simulink model "Aufiero_detumbling"  (R2021a)
settings: Solver=VariableStepAuto  StartTime=0.0  StopTime=250  FixedStep=1/262  RelTol=1e-3
settings Model: Creator=daniele.leuteri  LastModifiedBy=aufie
settings SolverCC: AlgebraicLoopSolver=TrustRegion
settings DebuggingCC: SFMachineParentedDataDiag=warning
settings SFSimCC: CustomCodeUndefinedFunction=UseInterfaceOnly

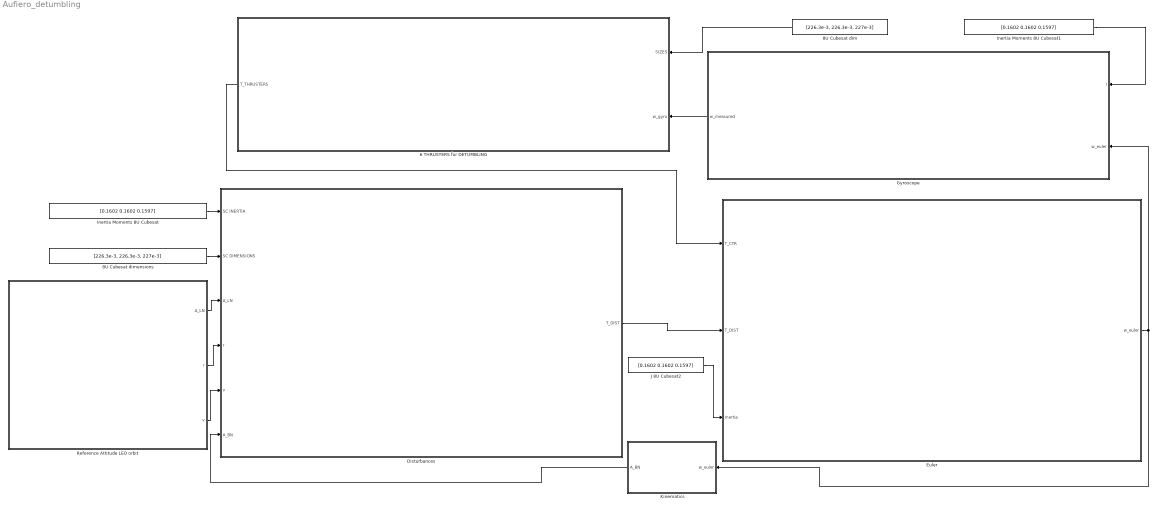
== system Aufiero_detumbling ==
  6 THRUSTERS for DETUMBLING : Subsystem
  8U Cubesat dim : Constant  Value=[226.3e-3, 226.3e-3, 227e-3]
  8U Cubesat dimensions : Constant  Value=[226.3e-3, 226.3e-3, 227e-3]
  Disturbances : Subsystem
  Euler : Subsystem
  Gyroscope : Subsystem
  Inertia Moments 8U Cubesat : Constant  Value=[0.1602 0.1602 0.1597]
  Inertia Moments 8U Cubesat1 : Constant  Value=[0.1602 0.1602 0.1597]
  J 8U Cubesat2 : Constant  Value=[0.1602 0.1602 0.1597]
  Kinematics : Subsystem
  Reference Attitude LEO orbit : Subsystem
  wires:
  8U Cubesat dimensions/1 -> Disturbances/2(SC DIMENSIONS)
  Reference Attitude LEO orbit/1(A_LN) -> Disturbances/3(A_LN)
  Reference Attitude LEO orbit/2(r) -> Disturbances/4(r)
  Reference Attitude LEO orbit/3(v) -> Disturbances/5(v)
  Inertia Moments 8U Cubesat/1 -> Disturbances/1(SC INERTIA)
  Kinematics/1(A_BN) -> Disturbances/6(A_BN)
  J 8U Cubesat2/1 -> Euler/3(Inertia)
  Disturbances/1(T_DIST) -> Euler/2(T_DIST)
  Inertia Moments 8U Cubesat1/1 -> Gyroscope/1(I)
  8U Cubesat dim/1 -> 6 THRUSTERS for DETUMBLING/1(SIZES)
  6 THRUSTERS for DETUMBLING/1(T_THRUSTERS) -> Euler/1(T_CTR)
  Gyroscope/1(w_measured) -> 6 THRUSTERS for DETUMBLING/2(w_gyro)
  Euler/1(w_euler) -> Kinematics/1(w_euler), Gyroscope/2(w_euler)

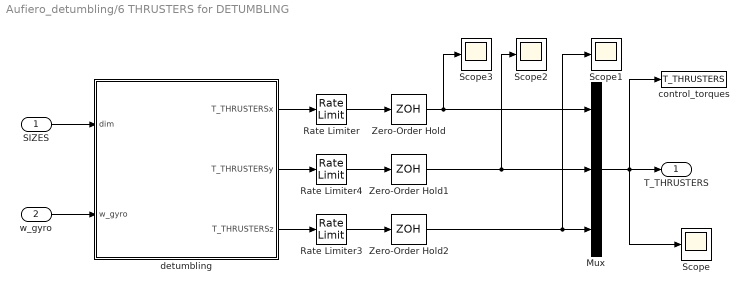
== system Aufiero_detumbling/6 THRUSTERS for DETUMBLING ==
  SIZES : Inport
  w_gyro : Inport  Port=2
  Mux : Mux  Inputs=3
  Rate Limiter : RateLimiter  RisingSlewLimit=1/0.1  FallingSlewLimit=-1/0.5  SampleTimeMode=inherited
  Rate Limiter3 : RateLimiter  RisingSlewLimit=1/0.1  FallingSlewLimit=-1/0.5  SampleTimeMode=inherited
  Rate Limiter4 : RateLimiter  RisingSlewLimit=1/0.1  FallingSlewLimit=-1/0.5  SampleTimeMode=inherited
  Scope{,1..3} (4 alike) : Scope
  Zero-Order Hold : ZeroOrderHold  SampleTime=0.05e-03
  Zero-Order Hold1 : ZeroOrderHold  SampleTime=0.05e-03
  Zero-Order Hold2 : ZeroOrderHold  SampleTime=0.05e-03
  control_torques : ToWorkspace  VariableName=T_THRUSTERS  SaveFormat=Timeseries  SampleTime=-1
  detumbling : MATLAB Function  TreatAsAtomicUnit=on
  T_THRUSTERS : Outport  VectorParamsAs1DForOutWhenUnconnected=off
  wires:
  SIZES/1 -> detumbling/1(dim)
  w_gyro/1 -> detumbling/2(w_gyro)
  Zero-Order Hold/1 -> Mux/1, Scope3/1
  Zero-Order Hold1/1 -> Mux/2, Scope2/1
  Zero-Order Hold2/1 -> Scope1/1, Mux/3
  Mux/1 -> control_torques/1, T_THRUSTERS/1, Scope/1
  detumbling/2(T_THRUSTERSy) -> Rate Limiter4/1
  detumbling/1(T_THRUSTERSx) -> Rate Limiter/1
  detumbling/3(T_THRUSTERSz) -> Rate Limiter3/1
  Rate Limiter/1 -> Zero-Order Hold/1
  Rate Limiter4/1 -> Zero-Order Hold1/1
  Rate Limiter3/1 -> Zero-Order Hold2/1

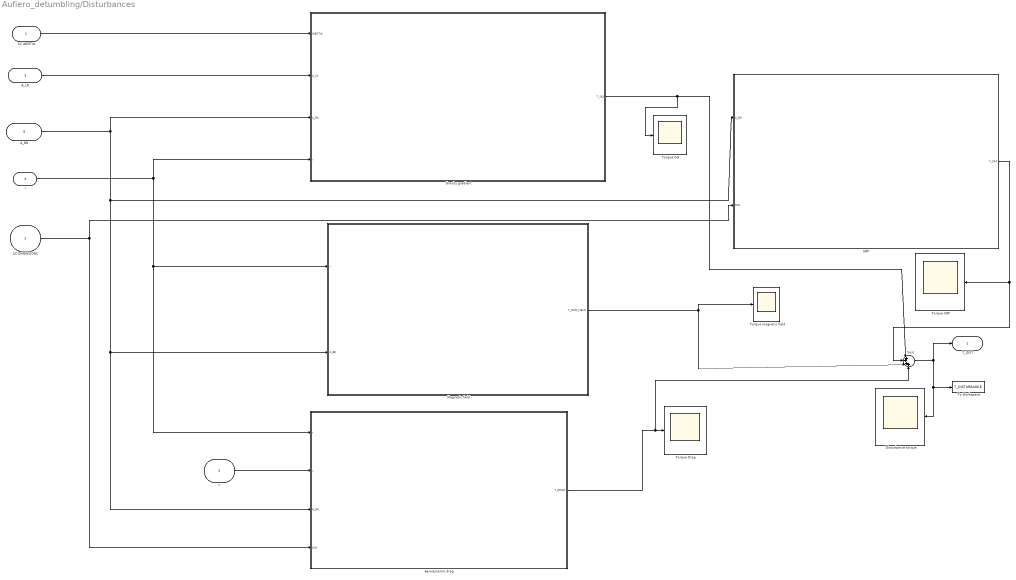
== system Aufiero_detumbling/Disturbances ==
  SC INERTIA : Inport
  SC DIMENSIONS : Inport  Port=2
  A_LN : Inport  Port=3
  r : Inport  Port=4
  v : Inport  Port=5
  A_BN : Inport  Port=6
  Aerodynamic drag : Subsystem
  Disturbance torque : Scope
  Gravity gradient : Subsystem
  Magnetic field : Subsystem
  SRP : Subsystem
  Sum : Sum  Inputs=|++++
  To Workspace : ToWorkspace  VariableName=T_DISTURBANCE  SaveFormat=Timeseries  SampleTime=-1
  Torque Drag : Scope
  Torque GG : Scope
  Torque SRP : Scope
  Torque magnetic field : Scope
  T_DIST : Outport  VectorParamsAs1DForOutWhenUnconnected=off
  wires:
  r/1 -> Gravity gradient/4(r), Aerodynamic drag/1(r), Magnetic field/1(r)
  v/1 -> Aerodynamic drag/2(v)
  A_BN/1 -> Gravity gradient/3(A_BN), Aerodynamic drag/3(A_BN), Magnetic field/2(A_BN), SRP/1(A_BN)
  SC DIMENSIONS/1 -> SRP/2(DIM), Aerodynamic drag/4(DIM)
  SC INERTIA/1 -> Gravity gradient/1(INERTIA)
  A_LN/1 -> Gravity gradient/2(A_LN)
  Gravity gradient/1(T_GG) -> Sum/1, Torque GG/1
  SRP/1(T_SRP) -> Sum/2, Torque SRP/1
  Aerodynamic drag/1(T_DRAG) -> Sum/4, Torque Drag/1
  Magnetic field/1(T_MAG_FIELD) -> Torque magnetic field/1, Sum/3
  Sum/1 -> Disturbance torque/1, To Workspace/1, T_DIST/1

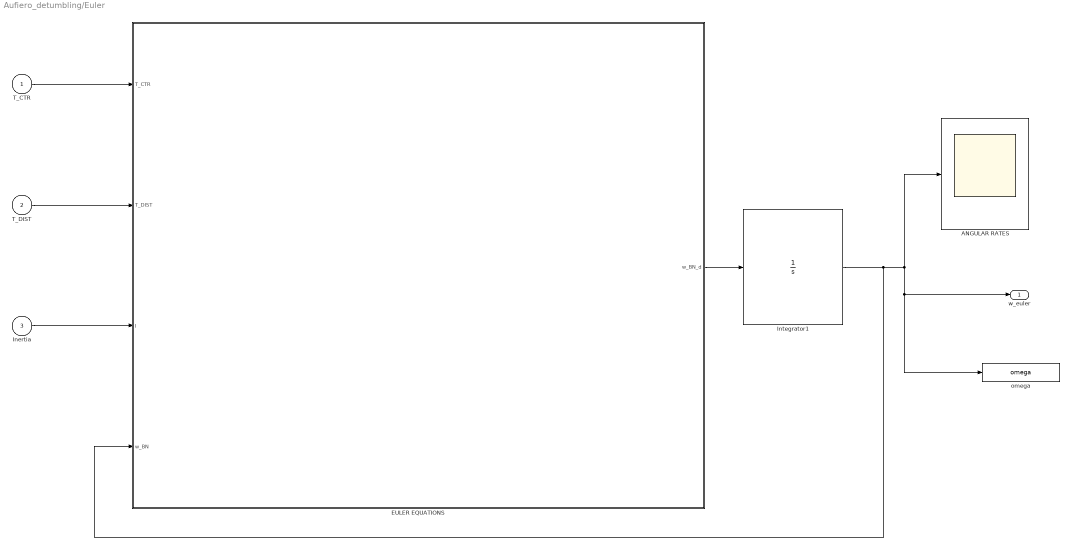
== system Aufiero_detumbling/Euler ==
  T_CTR : Inport
  T_DIST : Inport  Port=2
  Inertia : Inport  Port=3
  ANGULAR RATES : Scope
  EULER EQUATIONS : MATLAB Function  TreatAsAtomicUnit=on
  Integrator1 : Integrator  InitialCondition=[0.1 0.1 0.1]
  omega : ToWorkspace  VariableName=omega  SaveFormat=Timeseries  SampleTime=-1
  w_euler : Outport  VectorParamsAs1DForOutWhenUnconnected=off
  wires:
  T_CTR/1 -> EULER EQUATIONS/1(T_CTR)
  Inertia/1 -> EULER EQUATIONS/3(I)
  EULER EQUATIONS/1(w_BN_d) -> Integrator1/1
  T_DIST/1 -> EULER EQUATIONS/2(T_DIST)
  Integrator1/1 -> omega/1, w_euler/1, ANGULAR RATES/1, EULER EQUATIONS/4(w_BN)

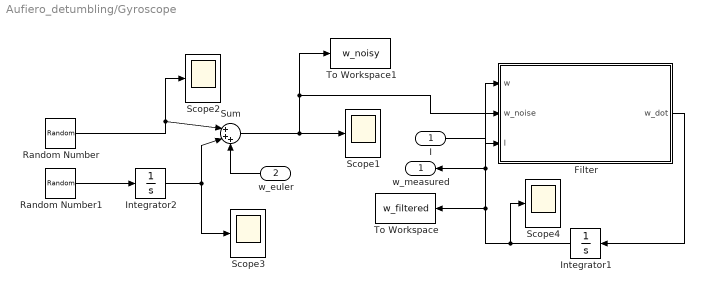
== system Aufiero_detumbling/Gyroscope ==
  I : Inport
  w_euler : Inport  Port=2
  "Filter " : MATLAB Function  TreatAsAtomicUnit=on
  Integrator1 : Integrator  InitialCondition=[0.1 0.1 0.1]
  Integrator2 : Integrator
  Random Number : RandomNumber  Variance=(0.15*pi/180/3600)*sqrt(1/262)  SampleTime=1/262
  Random Number1 : RandomNumber  Variance=(0.3*pi/180/3600)*sqrt(1/262)  SampleTime=1/262
  Scope{1..4} (4 alike) : Scope
  Sum : Sum  Inputs=|+++
  To Workspace : ToWorkspace  VariableName=w_filtered  SaveFormat=Timeseries  SampleTime=-1
  To Workspace1 : ToWorkspace  VariableName=w_noisy  SaveFormat=Timeseries  SampleTime=-1
  w_measured : Outport  VectorParamsAs1DForOutWhenUnconnected=off
  wires:
  Integrator1/1 -> Scope4/1, w_measured/1, "Filter "/1(w), To Workspace/1
  Random Number1/1 -> Integrator2/1
  Sum/1 -> To Workspace1/1, "Filter "/2(w_noise), Scope1/1
  Integrator2/1 -> Scope3/1, Sum/2
  Random Number/1 -> Scope2/1, Sum/1
  "Filter "/1(w_dot) -> Integrator1/1
  w_euler/1 -> Sum/3
  I/1 -> "Filter "/3(I)

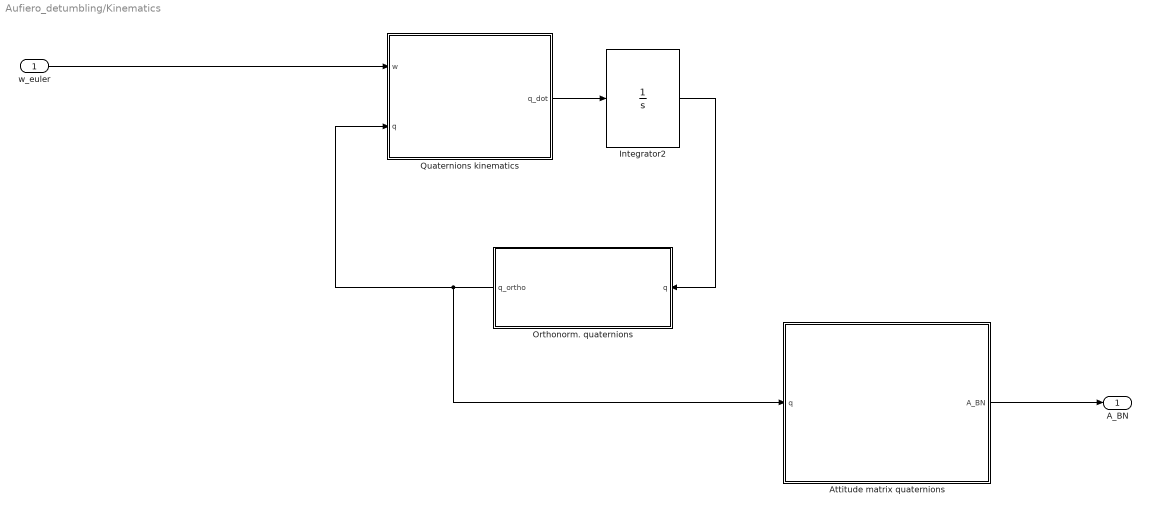
== system Aufiero_detumbling/Kinematics ==
  w_euler : Inport
  Attitude matrix quaternions : MATLAB Function  TreatAsAtomicUnit=on
  Integrator2 : Integrator  InitialCondition=[0 1/sqrt(3) 1/sqrt(3) 1/sqrt(3)]
  "Orthonorm. quaternions " : MATLAB Function  TreatAsAtomicUnit=on
  "Quaternions kinematics " : MATLAB Function  TreatAsAtomicUnit=on
  A_BN : Outport  VectorParamsAs1DForOutWhenUnconnected=off
  wires:
  w_euler/1 -> "Quaternions kinematics "/1(w)
  "Orthonorm. quaternions "/1(q_ortho) -> Attitude matrix quaternions/1(q), "Quaternions kinematics "/2(q)
  "Quaternions kinematics "/1(q_dot) -> Integrator2/1
  Attitude matrix quaternions/1(A_BN) -> A_BN/1
  Integrator2/1 -> "Orthonorm. quaternions "/1(q)

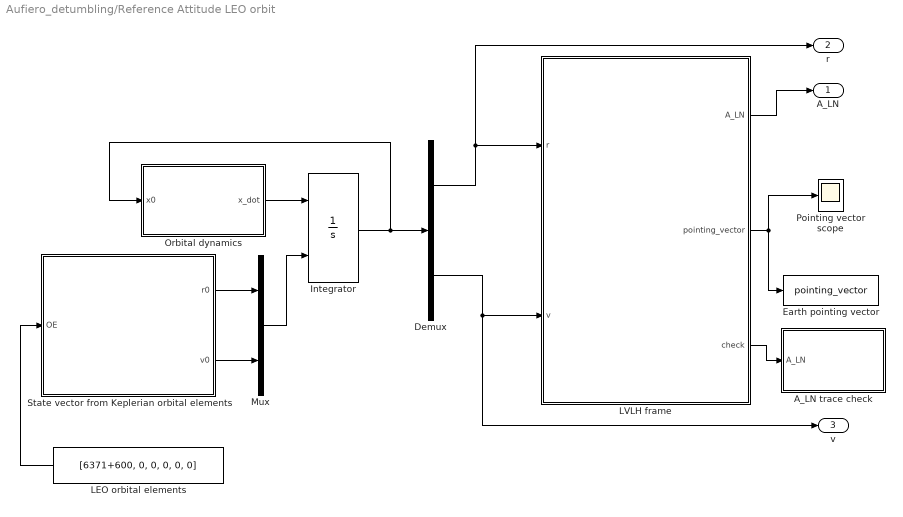
== system Aufiero_detumbling/Reference Attitude LEO orbit ==
  A_LN trace check : Subsystem
  Demux : Demux  Outputs=2
  Earth pointing vector : ToWorkspace  VariableName=pointing_vector  SampleTime=-1
  Integrator : Integrator  InitialConditionSource=external
  "LEO orbital elements " : Constant  Value=[6371+600, 0, 0, 0, 0, 0]
  LVLH frame : MATLAB Function  TreatAsAtomicUnit=on
  Mux : Mux  Inputs=2
  Orbital dynamics : MATLAB Function  TreatAsAtomicUnit=on
  Pointing vector scope : Scope
  State vector from Keplerian orbital elements : MATLAB Function  TreatAsAtomicUnit=on
  A_LN : Outport  VectorParamsAs1DForOutWhenUnconnected=off
  r : Outport  Port=2  VectorParamsAs1DForOutWhenUnconnected=off
  v : Outport  Port=3  VectorParamsAs1DForOutWhenUnconnected=off
  wires:
  LVLH frame/1(A_LN) -> A_LN/1
  Integrator/1 -> Demux/1, Orbital dynamics/1(x0)
  State vector from Keplerian orbital elements/2(v0) -> Mux/2
  Demux/2 -> v/1, LVLH frame/2(v)
  Demux/1 -> r/1, LVLH frame/1(r)
  Mux/1 -> Integrator/2
  Orbital dynamics/1(x_dot) -> Integrator/1
  State vector from Keplerian orbital elements/1(r0) -> Mux/1
  "LEO orbital elements "/1 -> State vector from Keplerian orbital elements/1(OE)
  LVLH frame/2(pointing_vector) -> Earth pointing vector/1, Pointing vector scope/1
  LVLH frame/3(check) -> A_LN trace check/1(A_LN)

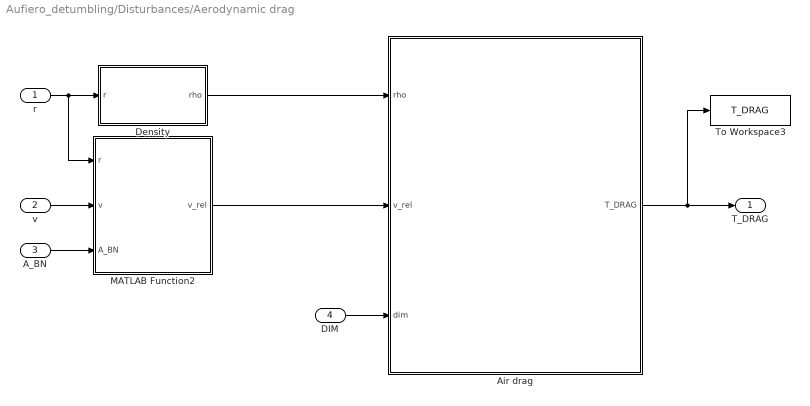
== system Aufiero_detumbling/Disturbances/Aerodynamic drag ==
  r : Inport
  v : Inport  Port=2
  A_BN : Inport  Port=3
  DIM : Inport  Port=4
  Air drag : MATLAB Function  TreatAsAtomicUnit=on
  Density : MATLAB Function  TreatAsAtomicUnit=on
  MATLAB Function2 : MATLAB Function  TreatAsAtomicUnit=on
  To Workspace3 : ToWorkspace  VariableName=T_DRAG  SaveFormat=Timeseries  SampleTime=-1
  T_DRAG : Outport  VectorParamsAs1DForOutWhenUnconnected=off
  wires:
  MATLAB Function2/1(v_rel) -> Air drag/2(v_rel)
  A_BN/1 -> MATLAB Function2/3(A_BN)
  Density/1(rho) -> Air drag/1(rho)
  v/1 -> MATLAB Function2/2(v)
  r/1 -> MATLAB Function2/1(r), Density/1(r)
  DIM/1 -> Air drag/3(dim)
  Air drag/1(T_DRAG) -> T_DRAG/1, To Workspace3/1

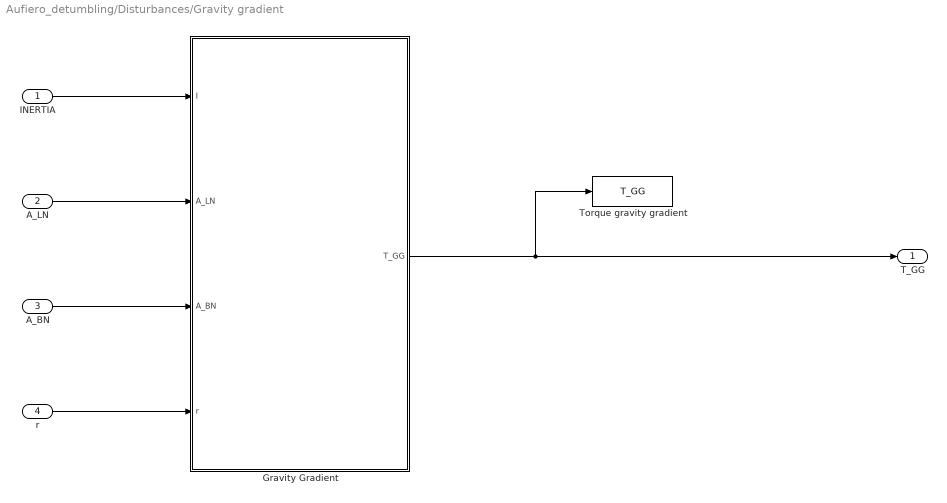
== system Aufiero_detumbling/Disturbances/Gravity gradient ==
  INERTIA : Inport
  A_LN : Inport  Port=2
  A_BN : Inport  Port=3
  r : Inport  Port=4
  Gravity Gradient : MATLAB Function  TreatAsAtomicUnit=on
  Torque gravity gradient : ToWorkspace  VariableName=T_GG  SaveFormat=Timeseries  SampleTime=-1
  T_GG : Outport  VectorParamsAs1DForOutWhenUnconnected=off
  wires:
  Gravity Gradient/1(T_GG) -> T_GG/1, Torque gravity gradient/1
  INERTIA/1 -> Gravity Gradient/1(I)
  A_LN/1 -> Gravity Gradient/2(A_LN)
  A_BN/1 -> Gravity Gradient/3(A_BN)
  r/1 -> Gravity Gradient/4(r)

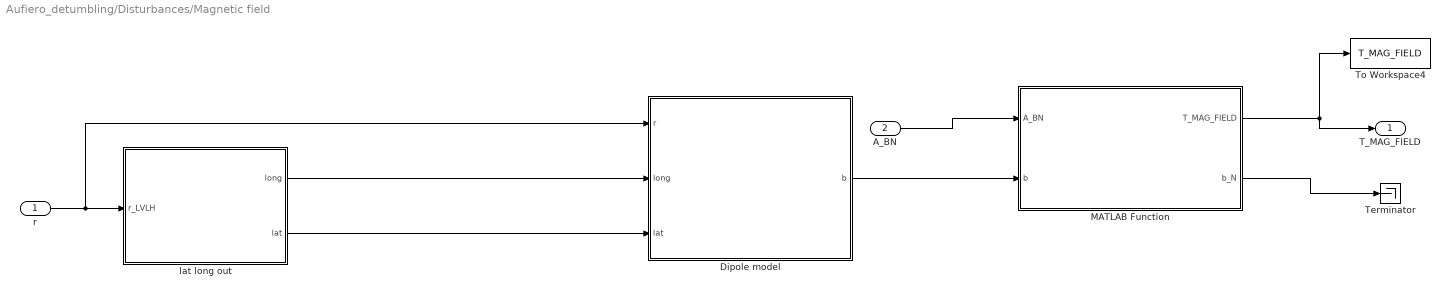
== system Aufiero_detumbling/Disturbances/Magnetic field ==
  r : Inport
  A_BN : Inport  Port=2
  Dipole model : MATLAB Function  TreatAsAtomicUnit=on
  MATLAB Function : MATLAB Function  TreatAsAtomicUnit=on
  Terminator : Terminator
  To Workspace4 : ToWorkspace  VariableName=T_MAG_FIELD  SaveFormat=Timeseries  SampleTime=-1
  "lat long out " : MATLAB Function  TreatAsAtomicUnit=on
  T_MAG_FIELD : Outport  VectorParamsAs1DForOutWhenUnconnected=off
  wires:
  r/1 -> Dipole model/1(r), "lat long out "/1(r_LVLH)
  A_BN/1 -> MATLAB Function/1(A_BN)
  Dipole model/1(b) -> MATLAB Function/2(b)
  MATLAB Function/1(T_MAG_FIELD) -> T_MAG_FIELD/1, To Workspace4/1
  MATLAB Function/2(b_N) -> Terminator/1
  "lat long out "/1(long) -> Dipole model/2(long)
  "lat long out "/2(lat) -> Dipole model/3(lat)

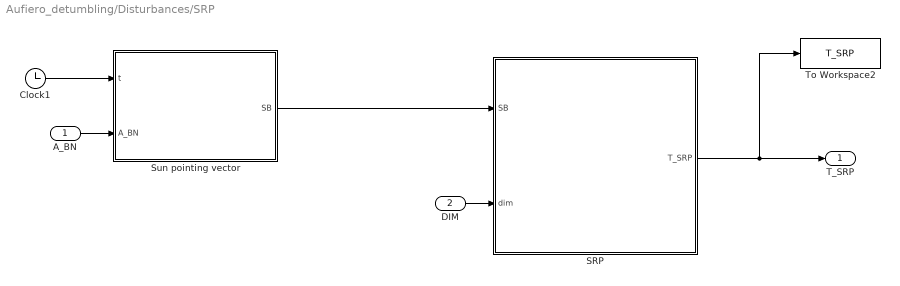
== system Aufiero_detumbling/Disturbances/SRP ==
  A_BN : Inport
  DIM : Inport  Port=2
  Clock1 : Clock
  SRP : MATLAB Function  TreatAsAtomicUnit=on
  Sun pointing vector : MATLAB Function  TreatAsAtomicUnit=on
  To Workspace2 : ToWorkspace  VariableName=T_SRP  SaveFormat=Timeseries  SampleTime=-1
  T_SRP : Outport  VectorParamsAs1DForOutWhenUnconnected=off
  wires:
  A_BN/1 -> Sun pointing vector/2(A_BN)
  DIM/1 -> SRP/2(dim)
  SRP/1(T_SRP) -> T_SRP/1, To Workspace2/1
  Clock1/1 -> Sun pointing vector/1(t)
  Sun pointing vector/1(SB) -> SRP/1(SB)

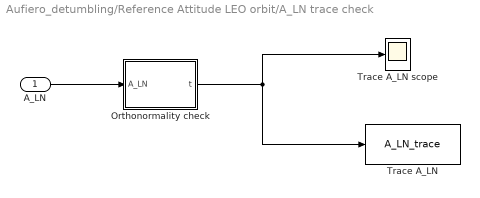
== system Aufiero_detumbling/Reference Attitude LEO orbit/A_LN trace check ==
  A_LN : Inport
  Orthonormality check : MATLAB Function  TreatAsAtomicUnit=on
  Trace A_LN : ToWorkspace  VariableName=A_LN_trace  SaveFormat=Timeseries  SampleTime=-1
  Trace A_LN scope : Scope
  wires:
  A_LN/1 -> Orthonormality check/1(A_LN)
  Orthonormality check/1(t) -> Trace A_LN scope/1, Trace A_LN/1

== matlab function Aufiero_detumbling/Disturbances/Aerodynamic drag/Density ==
  data: r input; rho output
function rho = exp_density_model(r)

r = norm(r);
h = (r - 6371000)*10^-3; % actual height [km]

if          h>=0 && h<25
            h_0 =   0; rho_0 =  1.225    ; H =   7.249;
    
elseif      h>=25 && h<30
            h_0 =   25; rho_0 = 3.899e-2 ; H =   6.349;
            
elseif      h>=30 && h<40
            h_0 =   30; rho_0 = 1.774e-2 ; H =   6.682;
                       
elseif      h>=40 && h<50
            h_0 =   40; rho_0 = 3.972e-3 ; H =   7.554;
            
elseif      h>=50 && h<60
            h_0 =   50; rho_0 = 1.057e-3 ; H =   8.382;
            
elseif      h>=60 && h<70
            h_0 =   60; rho_0 = 3.206e-4 ; H =   7.714;
            
elseif      h>=70 && h<80
            h_0 =   70; rho_0 = 8.770e-5 ; H =   6.549;

elseif      h>=80 && h<90
            h_0 =   80; rho_0 = 1.905e-5 ; H =   5.799;
            
elseif      h>=90 && h<100
            h_0 =   90; rho_0 = 3.396e-6 ; H =   5.382;
            
elseif      h>=100 && h<110
            h_0 =  100; rho_0 = 5.297e-7 ; H =   5.877;            
            
elseif      h>=110 && h<120
            h_0 =  110; rho_0 = 9.661e-8 ; H =   7.263;
            
elseif      h>=120 && h<130
            h_0 =  120; rho_0 = 2.438e-8 ; H =   9.473;           
            
elseif      h>=130 && h<140
            h_0 =  130; rho_0 = 8.484e-9 ; H =  12.636;
            
elseif      h>=140 && h<150
            h_0 =  140; rho_0 = 3.845e-9 ; H =  16.149;            
            
elseif      h>=150 && h<180
            h_0 =  150; rho_0 = 2.070e-9 ; H =  22.523;            
            
elseif      h>=180 && h<200
            h_0 =  180; rho_0 = 5.464e-10; H =  29.740;
            
elseif      h>=200 && h<250
            h_0 =  200; rho_0 = 2.789e-10; H =  37.105;            
            
elseif      h>=250 && h<300
            h_0 =  250; rho_0 = 7.248e-11; H =  45.546;            
            
elseif      h>=300 && h<350
            h_0 =  300; rho_0 = 2.418e-11; H =  53.628;
            
elseif      h>=350 && h<400
            h_0 =  350; rho_0 = 9.158e-12; H =  53.298;            
            
elseif      h>=400 && h<450
            h_0 =  400; rho_0 = 3.725e-12; H =  58.515;
            
elseif      h>=450 && h<500
            h_0 =  450; rho_0 = 1.585e-12; H =  60.828;
            
elseif      h>=500 && h<600
            h_0 =  500; rho_0 = 6.967e-13; H =  63.822;
            
elseif      h>=600 && h<700
            h_0 =  600; rho_0 = 1.454e-13; H =  71.835;            
            
elseif      h>=700 && h<800
            h_0 =  700; rho_0 = 3.614e-14; H =  88.667;            
            
elseif      h>=800 && h<900
            h_0 =  800; rho_0 = 1.170e-14; H = 124.64;
            
elseif      h>=900 && h<1000
            h_0 =  900; rho_0 = 5.245e-15; H = 181.05;                       
         
else      
            h_0 = 1000; rho_0 = 3.019e-15; H = 268.00;
            
end


rho = rho_0*exp(-(h-h_0)/H);

== matlab function Aufiero_detumbling/Disturbances/Aerodynamic drag/MATLAB Function2 ==
  data: r input; v_rel output; v input; A_BN input
function v_rel = relative_velocity(r,v,A_BN)

 % relative velocity between air and spacecraft
 
 v_rel = zeros (3,1);
 
 
 v_rel(1) = v(1) + 0.000072921*r(2);
 v_rel(2) = v(2) - 0.000072921*r(1);
 v_rel(3) = v(3);
 
 v_rel = A_BN * v_rel;
 
end

== matlab function Aufiero_detumbling/Euler/EULER EQUATIONS ==
  data: T_CTR input; T_DIST input; I input; w_BN input; w_BN_d output
function w_BN_d = euler (T_CTR, T_DIST, I, w_BN)

% EULER EQUATIONS INLCUDING DISTURBANCES AND CONTROL TORQUES

w_BN_d = zeros (1,3);

% DISTURBANCES + CONTROL TORQUE
w_BN_d(1) = (I(2)-I(3))/I(1)*w_BN(2)*w_BN(3) + T_DIST(1)/I(1) + T_CTR(1)/I(1);
w_BN_d(2) = (I(3)-I(1))/I(2)*w_BN(1)*w_BN(3) + T_DIST(2)/I(2) + T_CTR(2)/I(2);
w_BN_d(3) = (I(1)-I(2))/I(3)*w_BN(1)*w_BN(2) + T_DIST(3)/I(3) + T_CTR(3)/I(3);


w_BN_d = [w_BN_d(1) w_BN_d(2) w_BN_d(3)];


end

== matlab function Aufiero_detumbling/Kinematics/Attitude matrix quaternions ==
  data: q input; A_BN output
%function [A, ea_q] = quat_to_DCM(q)
function A_BN  = quat_to_DCM(q)

%% Elements of the A matrix as f(q)

A11 = q(1)^2 - q(2)^2 - q(3)^2 + q(4)^2;
A12 = 2*(q(1)*q(2) + q(3)*q(4));
A13 = 2*(q(1)*q(3) - q(2)*q(4));

A21 = 2*(q(1)*q(2) - q(3)*q(4));
A22 = -q(1)^2 + q(2)^2 - q(3)^2 + q(4)^2;
A23 = 2*(q(2)*q(3) + q(1)*q(4));

A31 = 2*(q(1)*q(3) + q(2)*q(4));
A32 = 2*(q(2)*q(3) - q(1)*q(4));
A33 = -q(1)^2 - q(2)^2 + q(3)^2 + q(4)^2;

A_BN = [ A11 A12 A13
      A21 A22 A23
      A31 A32 A33  ];

% %% New Euler Angles
% 
% phi = acosd(A(3,3));
% theta = -atand(A(3,1)/A(3,2));
% psi = atand(A(1,3)/A(2,3));
% 
% ea_q = [phi theta psi];

end

== matlab function Aufiero_detumbling/Disturbances/Magnetic field/Dipole model ==
  data: r input; long input; b output; lat input
function b = dipole_model(r, long, lat)

n_pole = [cos(80.37*pi/180)*cos(-72.62*pi/180);
          cos(80.37*pi/180)*sin(-72.62*pi/180);
                sin(80.37*pi/180)];
m_hat = -n_pole;

% Gaussian coefficients - IGRF 2015
g10 = -29442.0; %[nT]
g11 = -1501.0; %[nT]
h11 = 4797.1; %[nT]
H0 = sqrt(g10^2 + g11^2 + h11^2);
R_earth = 6371;

r_unit = [cos(lat*pi/180)*cos(long*pi/180);
    cos(lat*pi/180)*sin(long*pi/180);
    sin(lat*pi/180)];

b = (R_earth/norm(r))^3*H0*(3*dot(m_hat,r_unit)*r_unit - m_hat); %[nT]

end

== matlab function Aufiero_detumbling/Kinematics/Orthonorm. quaternions  ==
  data: q input; q_ortho output
function q_ortho = orho_quat(q)

Q1 = q(1)^2;
Q2 = q(2)^2;
Q3 = q(3)^2;
Q4 = q(4)^2;

Q = Q1 + Q2 + Q3 + Q4;

q_ortho = q/Q;

== matlab function Aufiero_detumbling/Kinematics/Quaternions kinematics  ==
  data: w input; q_dot output; q input
function q_dot = fcn(w, q)
% The input quaternions are already the orthonormalized ones

W = [   0   w(3)    -w(2)   w(1); 
      -w(3)  0       w(1)   w(2); 
       w(2) -w(1)     0     w(3); 
      -w(1) -w(2)   -w(3)    0   ];

q_dot = 0.5 * (W * q);

== matlab function Aufiero_detumbling/Disturbances/SRP/Sun pointing vector ==
  data: t input; SB output; A_BN input
function SB = sun_pointing(t, A_BN)

n = 2*pi/(365.25*3600*24); % Mean motion 
t0 = 0; % Initial time for the simulation 
eps = 23.45*pi/180; % Ecliptic inclination

% Sun pointing vector in inertial sun-centered reference frame
SN = [cos(n*t+t0); sin(n*t+t0)*cos(eps); sin(n*t+t0)*sin(eps)];

% Sun pointing vector in body frame
SB = A_BN * SN;

== matlab function Aufiero_detumbling/Disturbances/Magnetic field/lat long out  ==
  data: r_LVLH input; long output; lat output
function [long, lat] = ra_dec_from_r(r_LVLH)
% This function calculates the right ascension and the declination
% from the geocentric equatorial position vector.
%
% INPUT
%   r       position vector in ECI frame        [km]        [1x3]
%
% OUTPUT
%   ra      right ascension                     [deg]
%   dec     declination                         [deg]
%
%   Verified by Daniele Leuteri Costanzo

%% CALCULATE DIRECTION COSINES
l = r_LVLH(1)/norm(r_LVLH);
m = r_LVLH(2)/norm(r_LVLH);
n = r_LVLH(3)/norm(r_LVLH);

%% CALCULATE DECLINATION

lat = asind(n);

%% CALCULATE RIGHT ASCENSION

    if m > 0
        long = acosd(l/cosd(lat));
    else
        long = 360 - acosd(l/cosd(lat));
    end
end

== matlab function Aufiero_detumbling/Disturbances/Magnetic field/MATLAB Function ==
  data: A_BN input; T_MAG_FIELD output; b input; b_N output
function [T_MAG_FIELD, b_N] = magneticTorques(A_BN, b)

m_res = [0.1; 0.1; 0.1];

b_N = b*1e-9; %[T]

b_B = A_BN*b_N; %[T] magnetic field in the body frame

T_MAG_FIELD = cross(m_res,b_B); %[N.m]

end

== matlab function Aufiero_detumbling/Gyroscope/Filter  ==
  data: w input; w_dot output; w_noise input; I input
function w_dot = filter_gyro(w,w_noise, I)

k1 = 0.08;
I_x = I(1);
I_y = I(2);
I_z = I(3);

w_dot=zeros(3,1);
w_dot(1) =  ((I_y-I_z)/I_x)*w(2)*w(3) + k1 * (w_noise(1)-w(1));
w_dot(2) =  ((I_z-I_x)/I_y)*w(1)*w(3) + k1 * (w_noise(2)-w(2));
w_dot(3) =  ((I_x-I_y)/I_z)*w(1)*w(2) + k1 * (w_noise(3)-w(3));

== matlab function Aufiero_detumbling/Reference Attitude LEO orbit/Orbital dynamics ==
  data: x0 input; x_dot output
function x_dot  = twobodyproblem(x0)

mu = 398600;

% INPUT: STATE VECTOR

r = x0(1:3);  %[1x3] position
r_dot = x0(4:6);  %[1x3] velocity


% EQUIVALENT 1st ORDER SYSTEM

p_dot = r_dot'; % derivative of the position
v_dot = ((-mu/norm(r)^3).*r)'; % derivative of the velocity

% OUTPUT: DERIVATIVE OF THE STATE VECTOR

x_dot = [p_dot v_dot]';

end

== matlab function Aufiero_detumbling/Reference Attitude LEO orbit/State vector from Keplerian orbital elements ==
  data: OE input; r0 output; v0 output
function [r0,v0] = sv_from_oe (OE)
% This function computes the state vector (r,v) from the classical 
% orbital elements
%
% PROTOTYPE
%   [r,v] = sv_from_oe (OE, mu)
%
% INPUT
%
% OE        orbital elements [a e i W w TA]                             [1x6]       
% mu        gravitational parameter             [km^3/s^2]
%
% OUTPUT
% r         position vector in ECI frame        [km]                    [1x3]
% v         velocity vector in ECI frame        [km/s]                  [1x3]

mu = 398600;
% KEPLERIAN ORBITAL ELEMENTS
a = OE(1);
e = OE(2);
i = OE(3);
W = OE(4);
w = OE(5);
TA = OE(6);

% Semi latus rectum
p = a*(1 - norm(e)^2);

% Position and velocity in the perifocal frame

R = p/(1 + norm(e)*cos(TA));
rp = [R*cos(TA);R*sin(TA);0];
vp = [-sqrt(mu/p)*sin(TA); sqrt(mu/p)*(norm(e) + cos(TA)); 0];

% Rotation matrices
% R3_w - Rotation matrix about the z-axis through the angle w
% R1_i - Rotation matrix about the x-axis through the angle i
% R3_W - Rotation matrix about the z-axis through the angle W

R3_W = [ cos(W) sin(W) 0
        -sin(W) cos(W) 0
          0      0     1];
        
R1_i = [ 1     0       0
         0  cos(i) sin(i)
         0 -sin(i) cos(i)];
        
R3_w = [ cos(w) sin(w)   0
        -sin(w) cos(w)   0
            0       0    1];
       
% R_tot - Overall rotation from perifocal to geocentric equatorial frame
R_tot = R3_W' * R1_i' * R3_w';

% Position and velocity vectors expressed in the geocentric equatorial
% frame
r0 = R_tot*rp;
v0 = R_tot*vp;


end

== matlab function Aufiero_detumbling/Reference Attitude LEO orbit/LVLH frame ==
  data: r input; A_LN output; pointing_vector output; v input; check output
function [A_LN, pointing_vector, check]  = frame_tracking (r,v)
% Developing orthonormal frame to track
% r1 is the pointing vector (Earth pointing)

    r1 = r./norm(r);
    
    r3 = cross(r1,v)./norm(cross(r1,v));
    
    r2 = cross(r3,r1);
    
    pointing_vector = r1;
    
    A_LN = [r1' ; r2' ; r3'];
    
    check = trace(A_LN'*A_LN - eye(3));
  
end

== matlab function Aufiero_detumbling/6 THRUSTERS for DETUMBLING/detumbling ==
  data: dim input; w_gyro input; T_THRUSTERSx output; T_THRUSTERSy output; T_THRUSTERSz output
function [T_THRUSTERSx,T_THRUSTERSy,T_THRUSTERSz]  = control_detumbling (dim, w_gyro)

w_des = [0 0 0]';
w_err = w_gyro - w_des;

% On-off control
% 6 thrusters: 2 fixed in the +z axis, 4 for de-tumbling control

a = 15*pi/180; % deg
F = 25e-03; % N

eps = 1e-5;
l = dim(3)/2;
x1 = 0.2/2;
x2 = 0.09/2;

% Thruster configuration matrix
% T = [        l*F*sin(a)                 l*F*sin(a)                -l*F*sin(a)            -l*F*sin(a);
%             -l*F*cos(a)                 l*F*cos(a)                 l*F*cos(a)            -l*F*cos(a);
%      x1*F*sin(a) - x2*F*cos(a)    x1*F*cos(a) - x2*F*sin(a)     x1*F*sin(a)-x2*F*cos(a)   x1*F*cos(a)-x2*F*sin(a)];   
% 

T_max_1 = (2*l*F*sin(a));
T_max_2 = (2*l*F*cos(a));
T_max_3 = (2*(x1*F*cos(a)-x2*F*sin(a)));
T_max = diag([T_max_1;T_max_2;T_max_3]);

T_THRUSTERS = zeros(3,1);

for i = 1:3
     if (abs(w_err(i)) > eps)
         T_THRUSTERS(i) = - T_max(i,i) * sign(w_err(i)); 
     else
         T_THRUSTERS(i) = 0;
     end
 end


 T_THRUSTERSx = T_THRUSTERS(1);
 T_THRUSTERSy = T_THRUSTERS(2);
 T_THRUSTERSz = T_THRUSTERS(3);

== matlab function Aufiero_detumbling/Reference Attitude LEO orbit/A_LN trace check/Orthonormality check ==
  data: A_LN input; t output
function t = trace(A_LN)
% Checking orthonormality

tr_ALN = trace(eye(3)- A_LN.' * A_LN);

t = tr_ALN;

== matlab function Aufiero_detumbling/Disturbances/Gravity gradient/Gravity Gradient ==
  data: I input; T_GG output; A_LN input; A_BN input; r input
function T_GG = dist_gravity_gradient(I,A_LN, A_BN, r)
 
    mu = 398600; 
    R_earth = 6378;
    n = sqrt(mu/R_earth);
    
    
    A_BL = A_BN * A_LN';
    
    
    c = A_BL*[1;0;0];
    
    T_GG = zeros(1,3);
    
    T_GG(1) = (3 * n^2) * (I(3)-I(2)) * c(3) * c(2)/(I(1)*norm(r)^3);
    T_GG(2) = (3 * n^2) * (I(1)-I(3)) * c(1) * c(3)/(I(2)*norm(r)^3);
    T_GG(3) = (3 * n^2) * (I(2)-I(1)) * c(2) * c(1)/(I(3)*norm(r)^3);
    
end

== matlab function Aufiero_detumbling/Disturbances/SRP/SRP ==
  data: SB input; T_SRP output; dim input
function T_SRP = srp(SB, dim)

% Data
rho_d = 0.1;
rho_s = 0.5;

% Normals
n_1 = [1 0 0];
n_2 = [0 1 0];
n_3 = [0 0 1];
n_4 = [-1 0 0];
n_5 = [0 -1 0];
n_6 = [0 0 -1];

% 6U Cubesat sizes

w = dim(1); 
l = dim(2); 
h = dim(3); 

% Sections 
A_i_1 = w*l;
A_i_2 = w*h;
A_i_3 = l*h;
A_i_4 = A_i_1;
A_i_5 = A_i_2;
A_i_6 = A_i_3;

% Distance between the center of pressure and the center of mass

r_1 = [h/2 0.1 0.1];
r_2 = [0.2 l/2 0.2];
r_3 = [0.4 0.4 w/2];
r_4 = [-h/2 0.1 0.1];
r_5 = [0.2 -l/2 0.2];
r_6 = [0.4 0.4 -w/2];

% Compute Solar Radiation Pressure
% Data taken from Fundamentals of Spacecraft Attitude Determination and Control
solar_flux = 1362;        % W/m^2
c = 299792458;            % m/s
P = solar_flux/c;         % Pa

SB = SB';
   
    % Torque due to SRP, computed only on exposed surfaces.
    if dot(SB,n_1) >= 0
        F_srp_1 = P*A_i_1*dot(SB,n_1) * ((1-rho_s)*SB + (2*rho_s*dot(SB,n_1)+2/3*rho_d)*n_1);
        T_srp_1 = cross(r_1,F_srp_1);
    else
        T_srp_1 = [0 0 0];
    end
    
    if dot(SB,n_2) >= 0
        F_srp_2 = P*A_i_2*dot(SB,n_2) * ((1-rho_s)*SB + (2*rho_s*dot(SB,n_2)+2/3*rho_d)*n_2);
        T_srp_2 = cross(r_2,F_srp_2);
    else
        T_srp_2 = [0 0 0];
    end
    
    if dot(SB,n_3) >= 0
        F_srp_3 = P*A_i_3*dot(SB,n_3) * ((1-rho_s)*SB + (2*rho_s*dot(SB,n_3)+2/3*rho_d)*n_3);
        T_srp_3 = cross(r_3,F_srp_3);
    else
        T_srp_3 = [0 0 0];
    end
    
    if dot(SB,n_4) >= 0
        F_srp_4 = P*A_i_4*dot(SB,n_4) * ((1-rho_s)*SB + (2*rho_s*dot(SB,n_4)+2/3*rho_d)*n_4);
        T_srp_4 = cross(r_4,F_srp_4);
    else
        T_srp_4 = [0 0 0];
    end
    
    if dot(SB,n_5) >= 0
        F_srp_5 = P*A_i_5*dot(SB,n_5) * ((1-rho_s)*SB + (2*rho_s*dot(SB,n_5)+2/3*rho_d)*n_5);
        T_srp_5 = cross(r_5,F_srp_5);
    else
        T_srp_5 = [0 0 0];
    end
    
    if dot(SB,n_6) >= 0
        F_srp_6 = P*A_i_6*dot(SB,n_6) * ((1-rho_s)*SB + (2*rho_s*dot(SB,n_6)+2/3*rho_d)*n_6);
        T_aero_6 = cross(r_6,F_srp_6);
    else
        T_aero_6 = [0 0 0];
    end
    
    T_SRP = T_srp_1 + T_srp_2 + T_srp_3 + T_srp_4 + T_srp_5 + T_srp_5 + T_aero_6;
end

== matlab function Aufiero_detumbling/Disturbances/Aerodynamic drag/Air drag ==
  data: rho input; T_DRAG output; v_rel input; dim input
function T_DRAG = drag(rho,v_rel,dim)

air_dragT  = zeros(3,6);
air_dragF  = zeros(3,6);
cos_theta  = zeros(1,6);
T_DRAG = zeros(3,1); 

Cd = 2.2;

    % Normal to surfaces
    n = zeros(3,6);
    n(:,1) = [ 1  0  0 ]';
    n(:,2) = [ 0  1  0 ]';
    n(:,3) = [ 0  0  1 ]';
    n(:,4) = [-1  0  0 ]';
    n(:,5) = [ 0 -1  0 ]';
    n(:,6) = [ 0  0 -1 ]';
  
    b = zeros (3,6); % Offset mass centre - pressure centre
    b(:,1) = 0.1.*[    0    dim(2)  dim(3)]';
    b(:,2) = 0.1.*[ dim(1)     0    dim(3)]';
    b(:,3) = 0.1.*[ dim(1)   dim(2)    0  ]';
    b(:,4) = 0.1.*[    0    dim(2)  dim(3)]';
    b(:,5) = 0.1.*[ dim(1)     0    dim(3)]';
    b(:,6) = 0.1.*[ dim(1)   dim(2)    0  ]';
    
    % Area of surfaces
    A = zeros (6,1);
    A(1) = dim(3) * dim(2);
    A(4) = dim(3) * dim(2);
    A(2) = dim(3) * dim(1);
    A(5) = dim(3) * dim(1);
    A(3) = dim(2) * dim(1);
    A(6) = dim(2) * dim(1);
    
    
    
    for i = 1:6
        
        cos_theta(i) = dot(n(:,i),v_rel/norm(v_rel));
        
        if        cos_theta(i) < 0
                  air_dragT(:,i) = 0;
                  
                  
        
        else     
                
                  air_dragF = -0.5*rho*Cd*(norm(v_rel))^2*v_rel/norm(v_rel)*cos_theta(i)*A(i);
        
                  air_dragT(:,i) = cross(b(:,i),air_dragF);
                  
        end
        
    end
    
    T_DRAG = air_dragT(:,1) + air_dragT(:,2) + air_dragT(:,3) + air_dragT(:,4) + air_dragT(:,5) + air_dragT(:,6);
                 
                 
end
